simulink model "ex6"  (R2023b)
settings: Solver=ode3  StartTime=0.0  StopTime=inf  FixedStep=0.01  RelTol=1e-3
settings Model: Creator=alexm  LastModifiedBy=Andrei
settings OptimizationCC: ReuseModelBlockBuffer=off

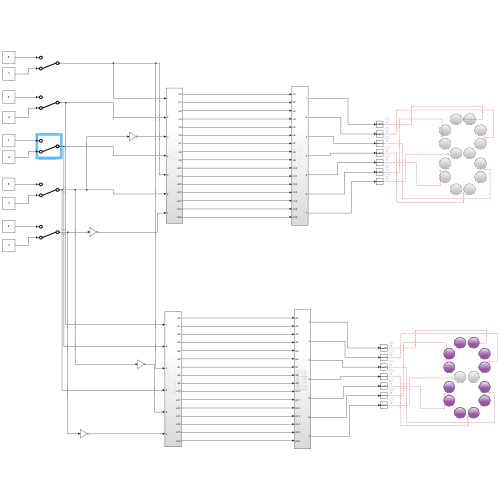
[thumbnail: Simulink's stored preview of the top-level diagram]
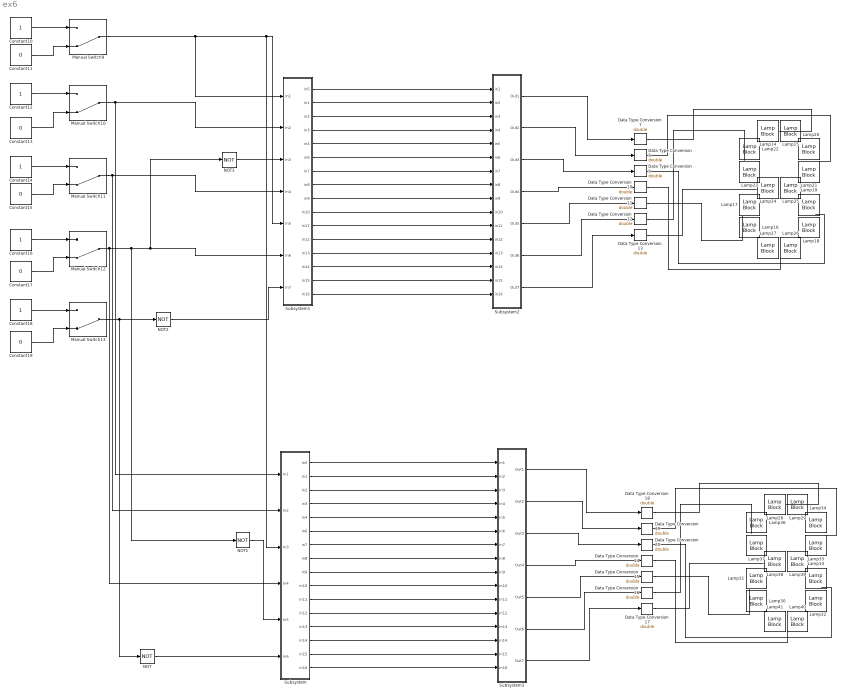
== system ex6 ==
  Constant{10,12,14,16,18} (5 alike) : Constant  OutDataTypeStr=double
  Constant{11,13,15,17,19} (5 alike) : Constant  Value=0  OutDataTypeStr=double
  Data Type Conversion{7..20} (14 alike) : DataTypeConversion  OutDataTypeStr=double  SaturateOnIntegerOverflow=off  RndMeth=Floor
  Lamp{14..41} (28 alike) : LampBlock  LabelPosition=Hide
  Manual Switch{9..13} (5 alike) : ManualSwitch  CurrentSetting=0
  NOT{,1..3} (4 alike) : Logic  Operator=NOT  IconShape=distinctive  AllPortsSameDT=off  OutDataTypeStr=boolean
  Subsystem : Subsystem
  Subsystem1 : Subsystem
  Subsystem2 : Subsystem
  Subsystem3 : Subsystem
  wires:
  Manual Switch13/1 -> NOT/1, NOT2/1
  Manual Switch12/1 -> Subsystem1/6(In6), NOT3/1, NOT1/1, Subsystem/4(In4)
  Manual Switch11/1 -> Subsystem1/4(In4), Subsystem/2(In2)
  Manual Switch10/1 -> Subsystem1/2(In2), Subsystem/1(In1)
  Manual Switch9/1 -> Subsystem1/5(In5), Subsystem/3(In3), Subsystem1/1(In1)
  Constant12/1 -> Manual Switch10/1
  Constant14/1 -> Manual Switch11/1
  Constant10/1 -> Manual Switch9/1
  Constant18/1 -> Manual Switch13/1
  Constant16/1 -> Manual Switch12/1
  Constant15/1 -> Manual Switch11/2
  Constant19/1 -> Manual Switch13/2
  Constant17/1 -> Manual Switch12/2
  Constant11/1 -> Manual Switch9/2
  Constant13/1 -> Manual Switch10/2
  NOT1/1 -> Subsystem/5(In5)
  NOT/1 -> Subsystem/6(In6)
  NOT3/1 -> Subsystem1/3(In3)
  NOT2/1 -> Subsystem1/7(In7)
  Subsystem1/16(in16) -> Subsystem2/16(in16)
  Subsystem1/15(in15) -> Subsystem2/15(in15)
  Subsystem1/14(in14) -> Subsystem2/14(in14)
  Subsystem1/13(in13) -> Subsystem2/13(in13)
  Subsystem1/12(in12) -> Subsystem2/12(in12)
  Subsystem1/11(in11) -> Subsystem2/11(in11)
  Subsystem1/10(in10) -> Subsystem2/10(in10)
  Subsystem1/9(in9) -> Subsystem2/9(in9)
  Subsystem1/8(in8) -> Subsystem2/8(in8)
  Subsystem1/7(in7) -> Subsystem2/7(in7)
  Subsystem1/6(in6) -> Subsystem2/6(in6)
  Subsystem1/1(in5) -> Subsystem2/1(in1)
  Subsystem1/2(in1) -> Subsystem2/2(in2)
  Subsystem1/3(in2) -> Subsystem2/3(in3)
  Subsystem1/4(in3) -> Subsystem2/4(in4)
  Subsystem1/5(in4) -> Subsystem2/5(in5)
  Data Type Conversion8/1 -> ?
  Data Type Conversion9/1 -> ?
  Data Type Conversion7/1 -> ?
  Data Type Conversion12/1 -> ?
  Data Type Conversion13/1 -> ?
  Data Type Conversion10/1 -> ?
  Subsystem2/6(Out6) -> Data Type Conversion12/1
  Subsystem2/7(Out7) -> Data Type Conversion13/1
  Subsystem2/1(Out1) -> Data Type Conversion7/1
  Subsystem2/4(Out4) -> Data Type Conversion10/1
  Subsystem2/2(Out2) -> Data Type Conversion8/1
  Subsystem2/3(Out3) -> Data Type Conversion9/1
  Subsystem2/5(Out5) -> Data Type Conversion11/1
  Data Type Conversion11/1 -> ?
  Subsystem/1(in5) -> Subsystem3/1(in1)
  Subsystem/2(in1) -> Subsystem3/2(in2)
  Subsystem/3(in2) -> Subsystem3/3(in3)
  Subsystem/4(in3) -> Subsystem3/4(in4)
  Subsystem/5(in4) -> Subsystem3/5(in5)
  Subsystem/6(in6) -> Subsystem3/6(in6)
  Subsystem/7(in7) -> Subsystem3/7(in7)
  Subsystem/8(in8) -> Subsystem3/8(in8)
  Subsystem/9(in9) -> Subsystem3/9(in9)
  Subsystem/10(in10) -> Subsystem3/10(in10)
  Subsystem/11(in11) -> Subsystem3/11(in11)
  Subsystem/12(in12) -> Subsystem3/12(in12)
  Subsystem/13(in13) -> Subsystem3/13(in13)
  Subsystem/14(in14) -> Subsystem3/14(in14)
  Subsystem/15(in15) -> Subsystem3/15(in15)
  Subsystem/16(in16) -> Subsystem3/16(in16)
  Data Type Conversion15/1 -> ?
  Data Type Conversion14/1 -> ?
  Data Type Conversion20/1 -> ?
  Data Type Conversion18/1 -> ?
  Data Type Conversion16/1 -> ?
  Data Type Conversion17/1 -> ?
  Subsystem3/5(Out5) -> Data Type Conversion15/1
  Subsystem3/6(Out6) -> Data Type Conversion16/1
  Subsystem3/7(Out7) -> Data Type Conversion17/1
  Subsystem3/3(Out3) -> Data Type Conversion20/1
  Subsystem3/2(Out2) -> Data Type Conversion19/1
  Subsystem3/1(Out1) -> Data Type Conversion18/1
  Subsystem3/4(Out4) -> Data Type Conversion14/1
  Data Type Conversion19/1 -> ?

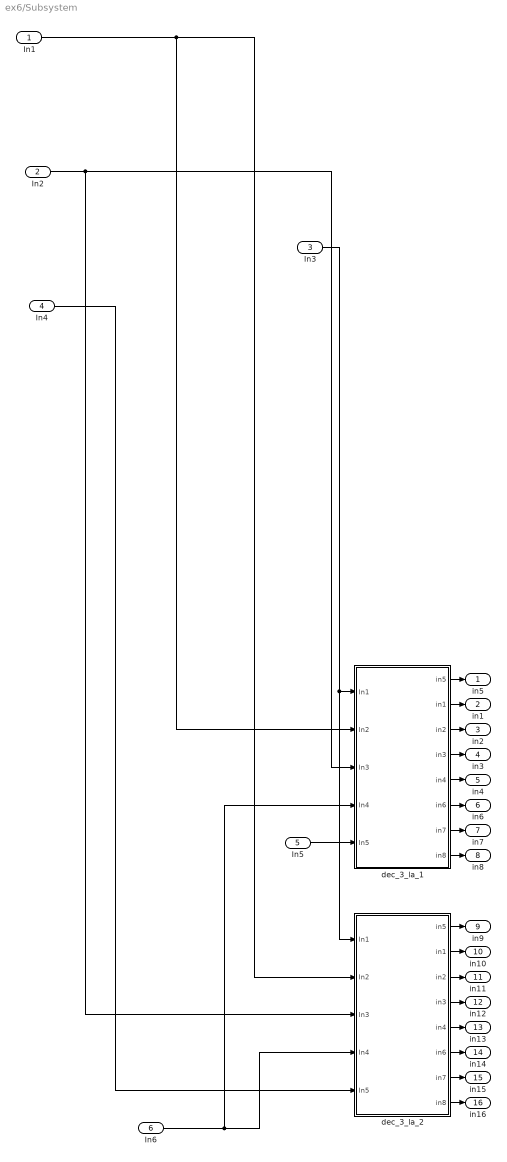
== system ex6/Subsystem ==
  In1 : Inport
  In2 : Inport  Port=2
  In3 : Inport  Port=3
  In4 : Inport  Port=4
  In5 : Inport  Port=5
  In6 : Inport  Port=6
  dec_3_la_1 : Subsystem
  dec_3_la_2 : Subsystem
  in5 : Outport
  in1 : Outport  Port=2
  in2 : Outport  Port=3
  in3 : Outport  Port=4
  in4 : Outport  Port=5
  in6 : Outport  Port=6
  in7 : Outport  Port=7
  in8 : Outport  Port=8
  in9 : Outport  Port=9
  in10 : Outport  Port=10
  in11 : Outport  Port=11
  in12 : Outport  Port=12
  in13 : Outport  Port=13
  in14 : Outport  Port=14
  in15 : Outport  Port=15
  in16 : Outport  Port=16
  wires:
  In2/1 -> dec_3_la_2/3(In3), dec_3_la_1/3(In3)
  In3/1 -> dec_3_la_2/1(In1), dec_3_la_1/1(In1)
  dec_3_la_1/3(in2) -> in2/1
  In6/1 -> dec_3_la_1/4(In4), dec_3_la_2/4(In4)
  In1/1 -> dec_3_la_2/2(In2), dec_3_la_1/2(In2)
  dec_3_la_2/8(in8) -> in16/1
  dec_3_la_2/7(in7) -> in15/1
  dec_3_la_1/7(in7) -> in7/1
  In5/1 -> dec_3_la_1/5(In5)
  dec_3_la_2/6(in6) -> in14/1
  dec_3_la_1/8(in8) -> in8/1
  dec_3_la_2/3(in2) -> in11/1
  In4/1 -> dec_3_la_2/5(In5)
  dec_3_la_2/4(in3) -> in12/1
  dec_3_la_2/5(in4) -> in13/1
  dec_3_la_1/1(in5) -> in5/1
  dec_3_la_1/5(in4) -> in4/1
  dec_3_la_1/6(in6) -> in6/1
  dec_3_la_1/4(in3) -> in3/1
  dec_3_la_1/2(in1) -> in1/1
  dec_3_la_2/2(in1) -> in10/1
  dec_3_la_2/1(in5) -> in9/1

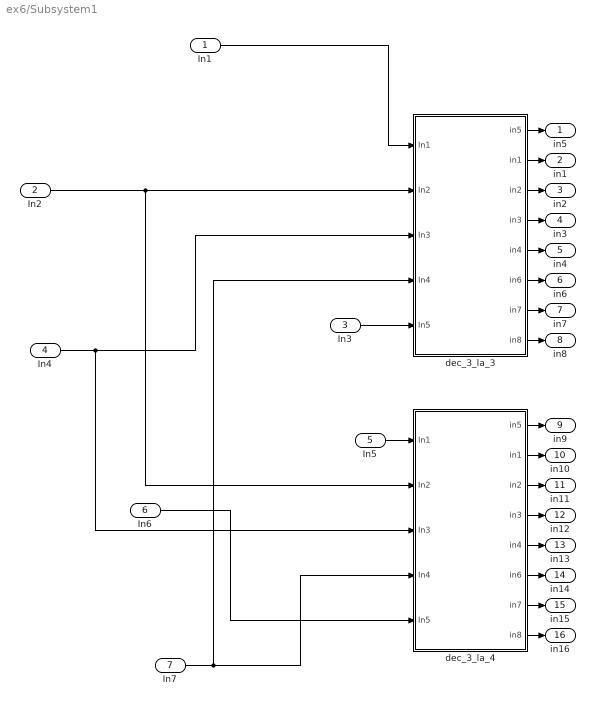
== system ex6/Subsystem1 ==
  In1 : Inport
  In2 : Inport  Port=2
  In3 : Inport  Port=3
  In4 : Inport  Port=4
  In5 : Inport  Port=5
  In6 : Inport  Port=6
  In7 : Inport  Port=7
  dec_3_la_3 : Subsystem
  dec_3_la_4 : Subsystem
  in5 : Outport
  in1 : Outport  Port=2
  in2 : Outport  Port=3
  in3 : Outport  Port=4
  in4 : Outport  Port=5
  in6 : Outport  Port=6
  in7 : Outport  Port=7
  in8 : Outport  Port=8
  in9 : Outport  Port=9
  in10 : Outport  Port=10
  in11 : Outport  Port=11
  in12 : Outport  Port=12
  in13 : Outport  Port=13
  in14 : Outport  Port=14
  in15 : Outport  Port=15
  in16 : Outport  Port=16
  wires:
  In2/1 -> dec_3_la_4/2(In2), dec_3_la_3/2(In2)
  dec_3_la_4/3(in2) -> in11/1
  dec_3_la_3/1(in5) -> in5/1
  In4/1 -> dec_3_la_4/3(In3), dec_3_la_3/3(In3)
  In7/1 -> dec_3_la_3/4(In4), dec_3_la_4/4(In4)
  In5/1 -> dec_3_la_4/1(In1)
  dec_3_la_4/7(in7) -> in15/1
  dec_3_la_4/1(in5) -> in9/1
  dec_3_la_4/2(in1) -> in10/1
  In6/1 -> dec_3_la_4/5(In5)
  dec_3_la_3/4(in3) -> in3/1
  dec_3_la_4/5(in4) -> in13/1
  dec_3_la_4/4(in3) -> in12/1
  In1/1 -> dec_3_la_3/1(In1)
  dec_3_la_4/6(in6) -> in14/1
  dec_3_la_3/2(in1) -> in1/1
  dec_3_la_4/8(in8) -> in16/1
  dec_3_la_3/3(in2) -> in2/1
  In3/1 -> dec_3_la_3/5(In5)
  dec_3_la_3/5(in4) -> in4/1
  dec_3_la_3/6(in6) -> in6/1
  dec_3_la_3/7(in7) -> in7/1
  dec_3_la_3/8(in8) -> in8/1

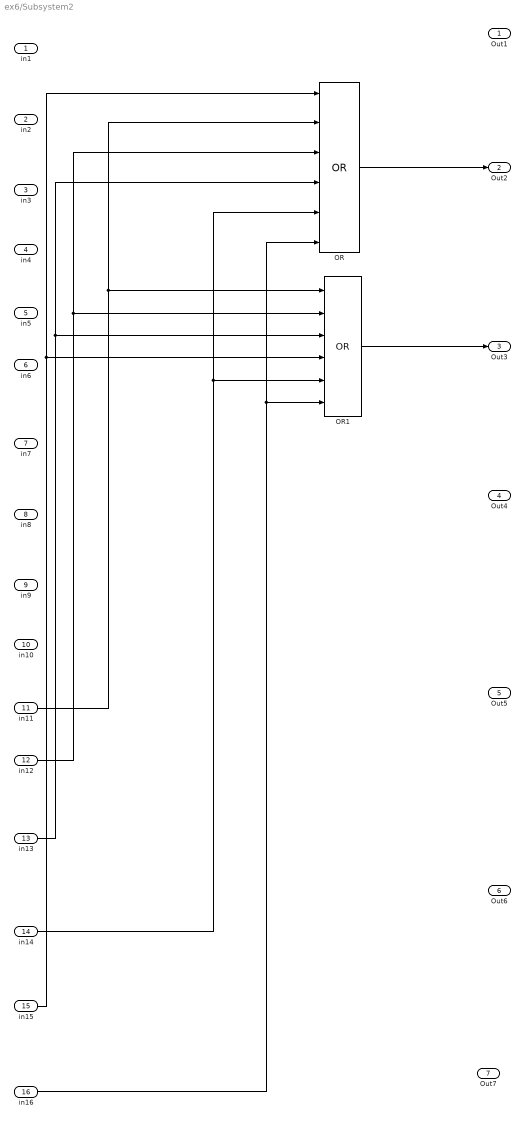
== system ex6/Subsystem2 ==
  in1 : Inport
  in2 : Inport  Port=2
  in3 : Inport  Port=3
  in4 : Inport  Port=4
  in5 : Inport  Port=5
  in6 : Inport  Port=6
  in7 : Inport  Port=7
  in8 : Inport  Port=8
  in9 : Inport  Port=9
  in10 : Inport  Port=10
  in11 : Inport  Port=11
  in12 : Inport  Port=12
  in13 : Inport  Port=13
  in14 : Inport  Port=14
  in15 : Inport  Port=15
  in16 : Inport  Port=16
  OR : Logic  Operator=OR  Inputs=6  IconShape=distinctive  AllPortsSameDT=off  OutDataTypeStr=boolean
  OR1 : Logic  Operator=OR  Inputs=6  IconShape=distinctive  AllPortsSameDT=off  OutDataTypeStr=boolean
  Out1 : Outport
  Out2 : Outport  Port=2
  Out3 : Outport  Port=3
  Out4 : Outport  Port=4
  Out5 : Outport  Port=5
  Out6 : Outport  Port=6
  Out7 : Outport  Port=7
  wires:
  OR/1 -> Out2/1
  in11/1 -> OR1/1, OR/2
  in12/1 -> OR1/2, OR/3
  in13/1 -> OR1/3, OR/4
  in14/1 -> OR1/5, OR/5
  in15/1 -> OR1/4, OR/1
  OR1/1 -> Out3/1
  in16/1 -> OR1/6, OR/6

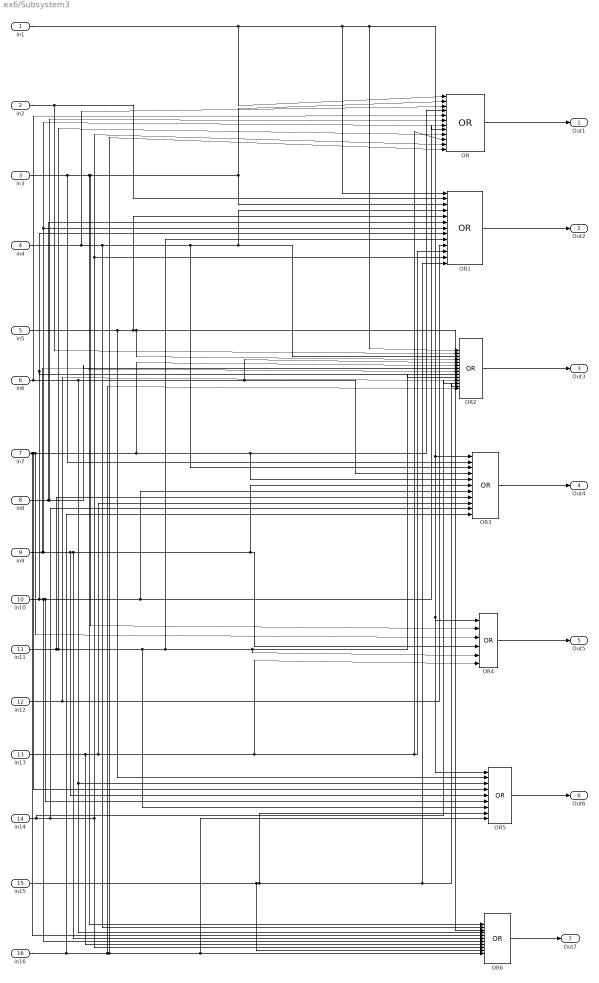
== system ex6/Subsystem3 ==
  in1 : Inport
  in2 : Inport  Port=2
  in3 : Inport  Port=3
  in4 : Inport  Port=4
  in5 : Inport  Port=5
  in6 : Inport  Port=6
  in7 : Inport  Port=7
  in8 : Inport  Port=8
  in9 : Inport  Port=9
  in10 : Inport  Port=10
  in11 : Inport  Port=11
  in12 : Inport  Port=12
  in13 : Inport  Port=13
  in14 : Inport  Port=14
  in15 : Inport  Port=15
  in16 : Inport  Port=16
  OR : Logic  Operator=OR  Inputs=12  IconShape=distinctive  AllPortsSameDT=off  OutDataTypeStr=boolean
  OR1 : Logic  Operator=OR  Inputs=13  IconShape=distinctive  AllPortsSameDT=off  OutDataTypeStr=boolean
  OR2 : Logic  Operator=OR  Inputs=14  IconShape=distinctive  AllPortsSameDT=off  OutDataTypeStr=boolean
  OR3 : Logic  Operator=OR  Inputs=11  IconShape=distinctive  AllPortsSameDT=off  OutDataTypeStr=boolean
  OR4 : Logic  Operator=OR  Inputs=6  IconShape=distinctive  AllPortsSameDT=off  OutDataTypeStr=boolean
  OR5 : Logic  Operator=OR  Inputs=9  IconShape=distinctive  AllPortsSameDT=off  OutDataTypeStr=boolean
  OR6 : Logic  Operator=OR  Inputs=11  IconShape=distinctive  AllPortsSameDT=off  OutDataTypeStr=boolean
  Out1 : Outport
  Out2 : Outport  Port=2
  Out3 : Outport  Port=3
  Out4 : Outport  Port=4
  Out5 : Outport  Port=5
  Out6 : Outport  Port=6
  Out7 : Outport  Port=7
  wires:
  in1/1 -> OR4/1, OR5/1, OR3/1, OR2/1, OR1/1, OR/1
  in3/1 -> OR1/3, OR/2, OR4/2, OR6/1, OR3/2
  in4/1 -> OR1/4, OR2/3, OR3/3, OR6/2, OR/3
  in7/1 -> OR/4, OR3/5, OR2/6, OR4/3, OR5/4, OR6/5
  in8/1 -> OR/6, OR2/7, OR1/6
  in9/1 -> OR3/6, OR4/4, OR6/6, OR5/5, OR/7, OR1/7, OR2/8
  in10/1 -> OR/8, OR3/7, OR5/6, OR6/7, OR1/8, OR2/9
  in11/1 -> OR2/10, OR4/5, OR1/9, OR5/7, OR/9, OR3/8
  in13/1 -> OR/10, OR1/11, OR4/6, OR3/9, OR6/8
  in14/1 -> OR/11, OR1/12, OR6/9, OR3/10, OR2/12
  OR/1 -> Out1/1
  OR1/1 -> Out2/1
  in2/1 -> OR2/2, OR1/2
  in5/1 -> OR6/3, OR2/4, OR1/5, OR5/2
  in12/1 -> OR1/10, OR2/11
  in15/1 -> OR1/13, OR2/13, OR5/8, OR6/10
  OR2/1 -> Out3/1
  OR3/1 -> Out4/1
  in16/1 -> OR5/9, OR6/11, OR/12, OR2/14, OR3/11
  OR4/1 -> Out5/1
  OR5/1 -> Out6/1
  OR6/1 -> Out7/1
  in6/1 -> OR6/4, OR5/3, OR2/5, OR3/4, OR/5

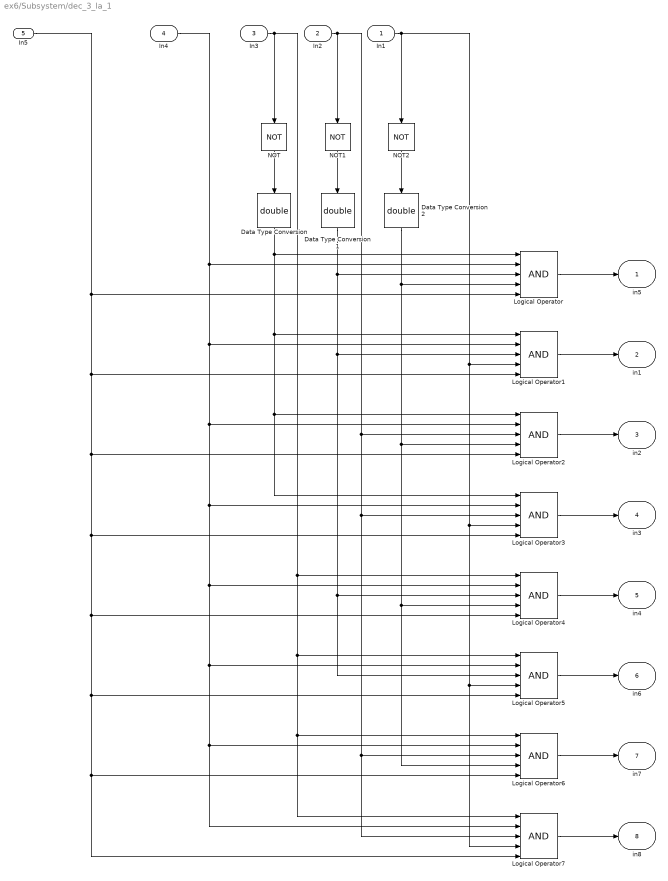
== system ex6/Subsystem/dec_3_la_1 ==
  In1 : Inport
  In2 : Inport  Port=2
  In3 : Inport  Port=3
  In4 : Inport  Description=n_G  Port=4
  In5 : Inport  Port=5
  Data Type Conversion : DataTypeConversion  OutDataTypeStr=double  SaturateOnIntegerOverflow=off  RndMeth=Floor
  Data Type Conversion1 : DataTypeConversion  OutDataTypeStr=double  SaturateOnIntegerOverflow=off  RndMeth=Floor
  Data Type Conversion2 : DataTypeConversion  OutDataTypeStr=double  SaturateOnIntegerOverflow=off  RndMeth=Floor
  Logical Operator{,1..7} (8 alike) : Logic  Inputs=5  IconShape=distinctive  AllPortsSameDT=off  OutDataTypeStr=boolean
  NOT : Logic  Operator=NOT  IconShape=distinctive  AllPortsSameDT=off  OutDataTypeStr=boolean
  NOT1 : Logic  Operator=NOT  IconShape=distinctive  AllPortsSameDT=off  OutDataTypeStr=boolean
  NOT2 : Logic  Operator=NOT  IconShape=distinctive  AllPortsSameDT=off  OutDataTypeStr=boolean
  in5 : Outport
  in1 : Outport  Port=2
  in2 : Outport  Port=3
  in3 : Outport  Port=4
  in4 : Outport  Port=5
  in6 : Outport  Port=6
  in7 : Outport  Port=7
  in8 : Outport  Port=8
  wires:
  In2/1 -> Logical Operator7/3, Logical Operator6/3, Logical Operator3/3, Logical Operator2/3, NOT1/1
  Data Type Conversion2/1 -> Logical Operator6/4, Logical Operator4/4, Logical Operator2/4, Logical Operator/4
  Data Type Conversion/1 -> Logical Operator3/1, Logical Operator2/1, Logical Operator1/1, Logical Operator/1
  In3/1 -> Logical Operator7/1, Logical Operator6/1, Logical Operator5/1, Logical Operator4/1, NOT/1
  Data Type Conversion1/1 -> Logical Operator5/3, Logical Operator4/3, Logical Operator1/3, Logical Operator/3
  In4/1 -> Logical Operator7/2, Logical Operator6/2, Logical Operator5/2, Logical Operator4/2, Logical Operator3/2, Logical Operator2/2, Logical Operator1/2, Logical Operator/2
  Logical Operator1/1 -> in1/1
  NOT/1 -> Data Type Conversion/1
  NOT1/1 -> Data Type Conversion1/1
  Logical Operator/1 -> in5/1
  Logical Operator5/1 -> in6/1
  Logical Operator3/1 -> in3/1
  Logical Operator4/1 -> in4/1
  Logical Operator2/1 -> in2/1
  In1/1 -> Logical Operator7/4, Logical Operator5/4, Logical Operator3/4, Logical Operator1/4, NOT2/1
  Logical Operator6/1 -> in7/1
  Logical Operator7/1 -> in8/1
  NOT2/1 -> Data Type Conversion2/1
  In5/1 -> Logical Operator6/5, Logical Operator7/5, Logical Operator5/5, Logical Operator4/5, Logical Operator3/5, Logical Operator2/5, Logical Operator1/5, Logical Operator/5

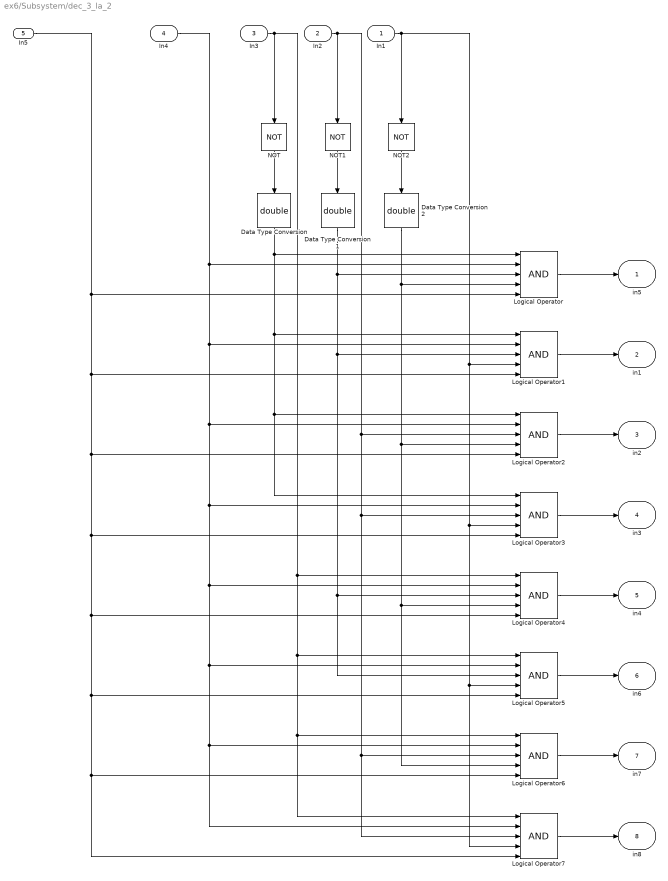
== system ex6/Subsystem/dec_3_la_2 ==
  In1 : Inport
  In2 : Inport  Port=2
  In3 : Inport  Port=3
  In4 : Inport  Port=4
  In5 : Inport  Port=5
  Data Type Conversion : DataTypeConversion  OutDataTypeStr=double  SaturateOnIntegerOverflow=off  RndMeth=Floor
  Data Type Conversion1 : DataTypeConversion  OutDataTypeStr=double  SaturateOnIntegerOverflow=off  RndMeth=Floor
  Data Type Conversion2 : DataTypeConversion  OutDataTypeStr=double  SaturateOnIntegerOverflow=off  RndMeth=Floor
  Logical Operator{,1..7} (8 alike) : Logic  Inputs=5  IconShape=distinctive  AllPortsSameDT=off  OutDataTypeStr=boolean
  NOT : Logic  Operator=NOT  IconShape=distinctive  AllPortsSameDT=off  OutDataTypeStr=boolean
  NOT1 : Logic  Operator=NOT  IconShape=distinctive  AllPortsSameDT=off  OutDataTypeStr=boolean
  NOT2 : Logic  Operator=NOT  IconShape=distinctive  AllPortsSameDT=off  OutDataTypeStr=boolean
  in5 : Outport
  in1 : Outport  Port=2
  in2 : Outport  Port=3
  in3 : Outport  Port=4
  in4 : Outport  Port=5
  in6 : Outport  Port=6
  in7 : Outport  Port=7
  in8 : Outport  Port=8
  wires:
  In2/1 -> Logical Operator7/3, Logical Operator6/3, Logical Operator3/3, Logical Operator2/3, NOT1/1
  Data Type Conversion2/1 -> Logical Operator6/4, Logical Operator4/4, Logical Operator2/4, Logical Operator/4
  Data Type Conversion/1 -> Logical Operator3/1, Logical Operator2/1, Logical Operator1/1, Logical Operator/1
  In3/1 -> Logical Operator7/1, Logical Operator6/1, Logical Operator5/1, Logical Operator4/1, NOT/1
  Data Type Conversion1/1 -> Logical Operator5/3, Logical Operator4/3, Logical Operator1/3, Logical Operator/3
  In4/1 -> Logical Operator7/2, Logical Operator6/2, Logical Operator5/2, Logical Operator4/2, Logical Operator3/2, Logical Operator2/2, Logical Operator1/2, Logical Operator/2
  Logical Operator1/1 -> in1/1
  NOT/1 -> Data Type Conversion/1
  NOT1/1 -> Data Type Conversion1/1
  Logical Operator/1 -> in5/1
  Logical Operator5/1 -> in6/1
  Logical Operator3/1 -> in3/1
  Logical Operator4/1 -> in4/1
  Logical Operator2/1 -> in2/1
  In1/1 -> Logical Operator7/4, Logical Operator5/4, Logical Operator3/4, Logical Operator1/4, NOT2/1
  Logical Operator6/1 -> in7/1
  Logical Operator7/1 -> in8/1
  NOT2/1 -> Data Type Conversion2/1
  In5/1 -> Logical Operator6/5, Logical Operator7/5, Logical Operator5/5, Logical Operator4/5, Logical Operator3/5, Logical Operator2/5, Logical Operator1/5, Logical Operator/5

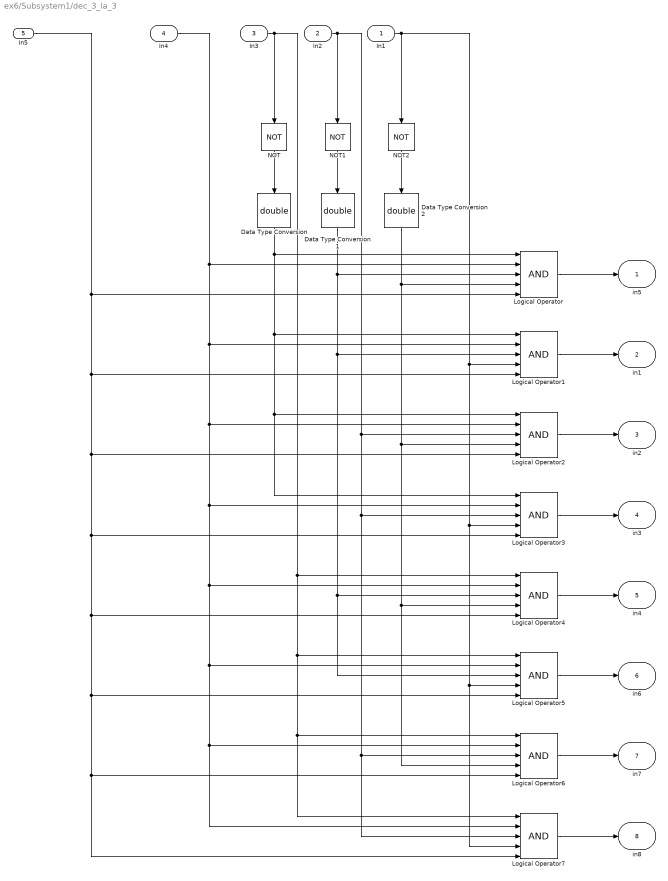
== system ex6/Subsystem1/dec_3_la_3 ==
  In1 : Inport
  In2 : Inport  Port=2
  In3 : Inport  Port=3
  In4 : Inport  Description=n_G  Port=4
  In5 : Inport  Port=5
  Data Type Conversion : DataTypeConversion  OutDataTypeStr=double  SaturateOnIntegerOverflow=off  RndMeth=Floor
  Data Type Conversion1 : DataTypeConversion  OutDataTypeStr=double  SaturateOnIntegerOverflow=off  RndMeth=Floor
  Data Type Conversion2 : DataTypeConversion  OutDataTypeStr=double  SaturateOnIntegerOverflow=off  RndMeth=Floor
  Logical Operator{,1..7} (8 alike) : Logic  Inputs=5  IconShape=distinctive  AllPortsSameDT=off  OutDataTypeStr=boolean
  NOT : Logic  Operator=NOT  IconShape=distinctive  AllPortsSameDT=off  OutDataTypeStr=boolean
  NOT1 : Logic  Operator=NOT  IconShape=distinctive  AllPortsSameDT=off  OutDataTypeStr=boolean
  NOT2 : Logic  Operator=NOT  IconShape=distinctive  AllPortsSameDT=off  OutDataTypeStr=boolean
  in5 : Outport
  in1 : Outport  Port=2
  in2 : Outport  Port=3
  in3 : Outport  Port=4
  in4 : Outport  Port=5
  in6 : Outport  Port=6
  in7 : Outport  Port=7
  in8 : Outport  Port=8
  wires:
  In2/1 -> Logical Operator7/3, Logical Operator6/3, Logical Operator3/3, Logical Operator2/3, NOT1/1
  Data Type Conversion2/1 -> Logical Operator6/4, Logical Operator4/4, Logical Operator2/4, Logical Operator/4
  Data Type Conversion/1 -> Logical Operator3/1, Logical Operator2/1, Logical Operator1/1, Logical Operator/1
  In3/1 -> Logical Operator7/1, Logical Operator6/1, Logical Operator5/1, Logical Operator4/1, NOT/1
  Data Type Conversion1/1 -> Logical Operator5/3, Logical Operator4/3, Logical Operator1/3, Logical Operator/3
  In4/1 -> Logical Operator7/2, Logical Operator6/2, Logical Operator5/2, Logical Operator4/2, Logical Operator3/2, Logical Operator2/2, Logical Operator1/2, Logical Operator/2
  Logical Operator1/1 -> in1/1
  NOT/1 -> Data Type Conversion/1
  NOT1/1 -> Data Type Conversion1/1
  Logical Operator/1 -> in5/1
  Logical Operator5/1 -> in6/1
  Logical Operator3/1 -> in3/1
  Logical Operator4/1 -> in4/1
  Logical Operator2/1 -> in2/1
  In1/1 -> Logical Operator7/4, Logical Operator5/4, Logical Operator3/4, Logical Operator1/4, NOT2/1
  Logical Operator6/1 -> in7/1
  Logical Operator7/1 -> in8/1
  NOT2/1 -> Data Type Conversion2/1
  In5/1 -> Logical Operator6/5, Logical Operator7/5, Logical Operator5/5, Logical Operator4/5, Logical Operator3/5, Logical Operator2/5, Logical Operator1/5, Logical Operator/5

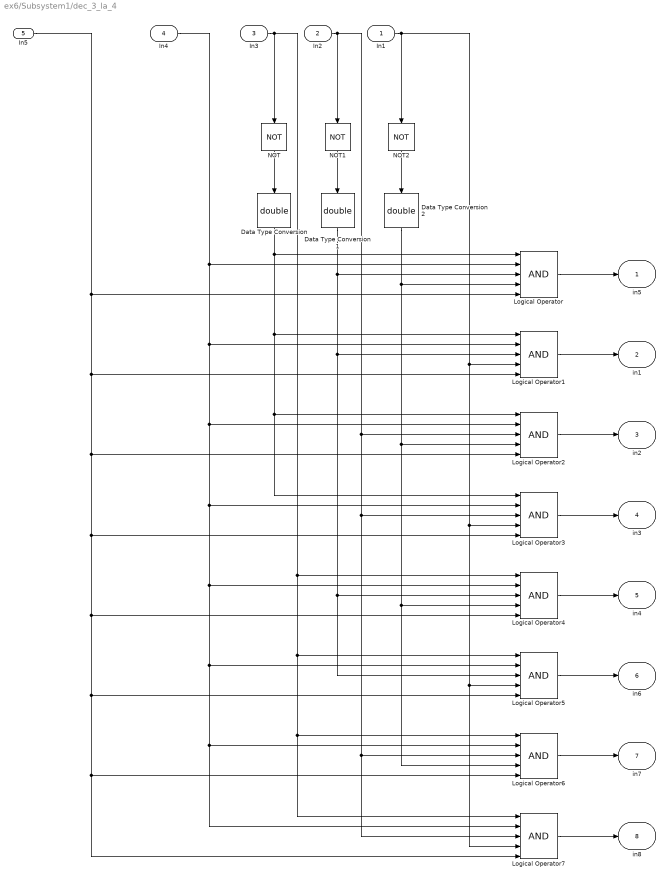
== system ex6/Subsystem1/dec_3_la_4 ==
  In1 : Inport
  In2 : Inport  Port=2
  In3 : Inport  Port=3
  In4 : Inport  Port=4
  In5 : Inport  Port=5
  Data Type Conversion : DataTypeConversion  OutDataTypeStr=double  SaturateOnIntegerOverflow=off  RndMeth=Floor
  Data Type Conversion1 : DataTypeConversion  OutDataTypeStr=double  SaturateOnIntegerOverflow=off  RndMeth=Floor
  Data Type Conversion2 : DataTypeConversion  OutDataTypeStr=double  SaturateOnIntegerOverflow=off  RndMeth=Floor
  Logical Operator{,1..7} (8 alike) : Logic  Inputs=5  IconShape=distinctive  AllPortsSameDT=off  OutDataTypeStr=boolean
  NOT : Logic  Operator=NOT  IconShape=distinctive  AllPortsSameDT=off  OutDataTypeStr=boolean
  NOT1 : Logic  Operator=NOT  IconShape=distinctive  AllPortsSameDT=off  OutDataTypeStr=boolean
  NOT2 : Logic  Operator=NOT  IconShape=distinctive  AllPortsSameDT=off  OutDataTypeStr=boolean
  in5 : Outport
  in1 : Outport  Port=2
  in2 : Outport  Port=3
  in3 : Outport  Port=4
  in4 : Outport  Port=5
  in6 : Outport  Port=6
  in7 : Outport  Port=7
  in8 : Outport  Port=8
  wires:
  In2/1 -> Logical Operator7/3, Logical Operator6/3, Logical Operator3/3, Logical Operator2/3, NOT1/1
  Data Type Conversion2/1 -> Logical Operator6/4, Logical Operator4/4, Logical Operator2/4, Logical Operator/4
  Data Type Conversion/1 -> Logical Operator3/1, Logical Operator2/1, Logical Operator1/1, Logical Operator/1
  In3/1 -> Logical Operator7/1, Logical Operator6/1, Logical Operator5/1, Logical Operator4/1, NOT/1
  Data Type Conversion1/1 -> Logical Operator5/3, Logical Operator4/3, Logical Operator1/3, Logical Operator/3
  In4/1 -> Logical Operator7/2, Logical Operator6/2, Logical Operator5/2, Logical Operator4/2, Logical Operator3/2, Logical Operator2/2, Logical Operator1/2, Logical Operator/2
  Logical Operator1/1 -> in1/1
  NOT/1 -> Data Type Conversion/1
  NOT1/1 -> Data Type Conversion1/1
  Logical Operator/1 -> in5/1
  Logical Operator5/1 -> in6/1
  Logical Operator3/1 -> in3/1
  Logical Operator4/1 -> in4/1
  Logical Operator2/1 -> in2/1
  In1/1 -> Logical Operator7/4, Logical Operator5/4, Logical Operator3/4, Logical Operator1/4, NOT2/1
  Logical Operator6/1 -> in7/1
  Logical Operator7/1 -> in8/1
  NOT2/1 -> Data Type Conversion2/1
  In5/1 -> Logical Operator6/5, Logical Operator7/5, Logical Operator5/5, Logical Operator4/5, Logical Operator3/5, Logical Operator2/5, Logical Operator1/5, Logical Operator/5
